simulink model "plant"  (R2025b)
settings: Solver=ode4  StartTime=0.0  StopTime=10.0  FixedStep=Ts_inner  RelTol=1e-3
undefined symbols (not defined in the file): quadcop, Ts_gcs
libraries: matrix_library x1
settings Model: DataDictionary=project.sldd  Creator=Nick  LastModifiedBy=Rakete

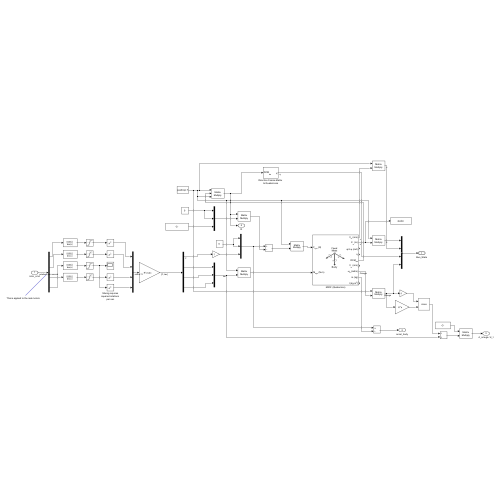
[thumbnail: Simulink's stored preview of the top-level diagram]
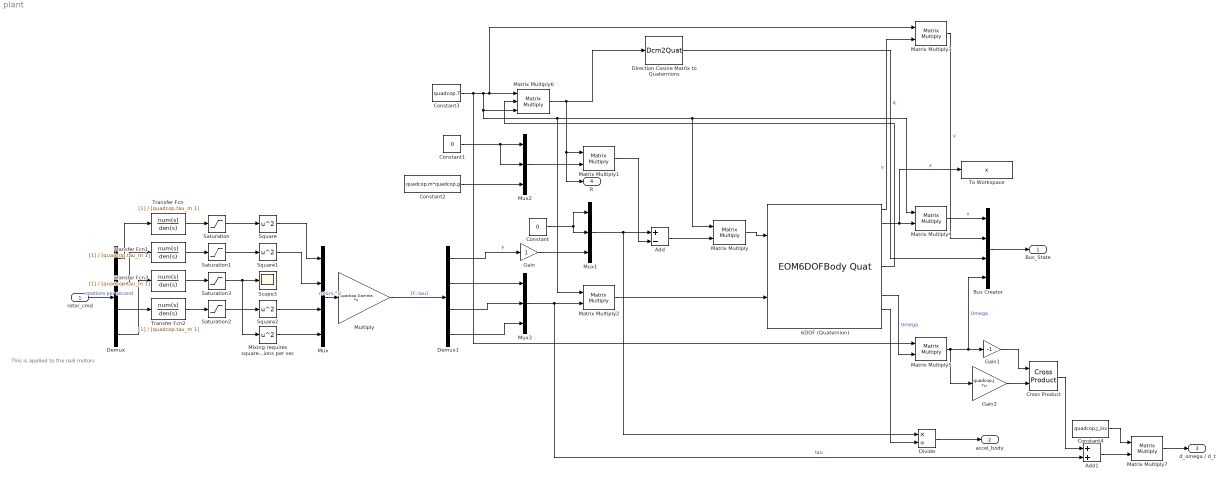
== system plant ==
  note: This is applied to the real motors
  rotor_cmd : Inport
  6DOF (Quaternion) : EOM6DOFBodyQuat  xme_0=quadcop.x0  Vm_0=quadcop.v0  eul_0=quadcop.euler0  pm_0=quadcop.w0  mass_0=quadcop.m  inertia=quadcop.J  mass_flag=on
  Add : Sum  Inputs=+-
  Add1 : Sum
  Bus Creator : BusCreator  Inputs=4  OutDataTypeStr=Bus: Bus_State  NonVirtualBus=on
  Constant : Constant  Value=0
  Constant1 : Constant  Value=0
  Constant2 : Constant  Value=quadcop.m*quadcop.g
  Constant3 : Constant  Value=quadcop.T
  Constant4 : Constant  Value=quadcop.J_inv
  Cross Product : matrix_library/Cross Product
  Demux : Demux
  Demux1 : Demux
  Direction Cosine Matrix to Quaternions : Dcm2Quat
  Divide : Product  Inputs=*/
  Gain : Gain
  Gain1 : Gain  Gain=-1
  Gain2 : Gain  Gain=quadcop.J  Multiplication=Matrix(K*u)
  Matrix Multiply{,1..5,7} (7 alike) : Product  Multiplication=Matrix(*)
  Matrix Multiply6 : Product  Inputs=3  Multiplication=Matrix(*)
  Mixing requires squared rotations per sec : Math  Operator=square
  Multiply : Gain  Gain=quadcop.Gamma  Multiplication=Matrix(K*u) (u vector)
  Mux : Mux
  Mux1 : Mux  Inputs=3
  Mux2 : Mux  Inputs=3
  Mux3 : Mux  Inputs=3
  Saturation{,1..3} (4 alike) : Saturate  UpperLimit=quadcop.rotors_max  LowerLimit=quadcop.rotors_min
  Scope3 : Scope
      settings: ActiveDisplayYMinimum=-6.46825029253925  ActiveDisplayYMaximum=58.214252632853267  DataLoggingVariableName=ScopeData3
  Square : Math  Operator=square
  Square1 : Math  Operator=square
  Square2 : Math  Operator=square
  To Workspace : ToWorkspace  VariableName=x  SaveFormat=Timeseries  SampleTime=Ts_gcs
  Transfer Fcn{,1..3} (4 alike) : TransferFcn  Denominator=[quadcop.tau_m 1]
  Bus_State : Outport  OutDataTypeStr=Bus: Bus_State
  accel_body : Outport  Port=2
  d_omega / d_t : Outport  Port=3
  R : Outport  Port=4
  wires:
  rotor_cmd/1 -> Demux/1  "rotations per second"
  Divide/1 -> accel_body/1
  Mux3/1 -> Add1/2, Matrix Multiply2/2  "tau"
  Transfer Fcn/1 -> Saturation/1
  6DOF (Quaternion)/8 -> Divide/2
  Mux/1 -> Multiply/1  "rotors.^2"
  Demux/1 -> Transfer Fcn/1
  Cross Product/1 -> Add1/1
  6DOF (Quaternion)/5 -> Matrix Multiply6/2
  Transfer Fcn1/1 -> Saturation1/1
  Demux/2 -> Transfer Fcn1/1
  Demux/3 -> Transfer Fcn2/1
  Demux/4 -> Transfer Fcn3/1
  Transfer Fcn3/1 -> Saturation3/1
  Gain1/1 -> Cross Product/1
  Transfer Fcn2/1 -> Saturation2/1
  6DOF (Quaternion)/7 -> Matrix Multiply5/2  "Omega"
  Saturation/1 -> Square/1
  Saturation1/1 -> Square1/1
  Saturation3/1 -> Scope3/1, Mixing requires squared rotations per sec/1
  Add/1 -> Matrix Multiply/2
  Saturation2/1 -> Square2/1
  Constant/1 -> Mux1/2, Mux1/1
  Square/1 -> Mux/1
  Square1/1 -> Mux/2
  Constant3/1 -> Matrix Multiply4/1, Matrix Multiply/1, Matrix Multiply2/1, Matrix Multiply6/3, Matrix Multiply3/1, Matrix Multiply6/1, Matrix Multiply5/1
  Square2/1 -> Mux/3
  Matrix Multiply/1 -> 6DOF (Quaternion)/1
  Mixing requires squared rotations per sec/1 -> Mux/4
  Multiply/1 -> Demux1/1  "[F; tau]"
  Gain/1 -> Mux1/3
  Constant1/1 -> Mux2/1, Mux2/2
  Mux2/1 -> Matrix Multiply1/2
  Constant2/1 -> Mux2/3
  Mux1/1 -> Add/1, Divide/1
  Demux1/1 -> Gain/1  "F"
  Demux1/2 -> Mux3/1
  Demux1/3 -> Mux3/2
  Add1/1 -> Matrix Multiply7/2
  Demux1/4 -> Mux3/3
  Matrix Multiply6/1 -> R/1, Matrix Multiply1/1, Direction Cosine Matrix to Quaternions/1
  Matrix Multiply1/1 -> Add/2
  Matrix Multiply2/1 -> 6DOF (Quaternion)/2
  Direction Cosine Matrix to Quaternions/1 -> Bus Creator/3  "q"
  Constant4/1 -> Matrix Multiply7/1
  Gain2/1 -> Cross Product/2
  6DOF (Quaternion)/1 -> Matrix Multiply3/2  "v"
  6DOF (Quaternion)/2 -> To Workspace/1, Matrix Multiply4/2  "x"
  Matrix Multiply3/1 -> Bus Creator/2  "v"
  Matrix Multiply4/1 -> Bus Creator/1  "x"
  Matrix Multiply5/1 -> Bus Creator/4, Gain1/1, Gain2/1  "Omega"
  Bus Creator/1 -> Bus_State/1
  Matrix Multiply7/1 -> d_omega / d_t/1
